simulink model "SystemPIDOpenLoopTest"  (Simulink 7.7)
settings: Solver=ode4  StartTime=0.0  StopTime=50  FixedStep=0.01  RelTol=1e-3
libraries: simulink x4
settings Model: Creator=Rakhi  LastModifiedBy=Rakhi

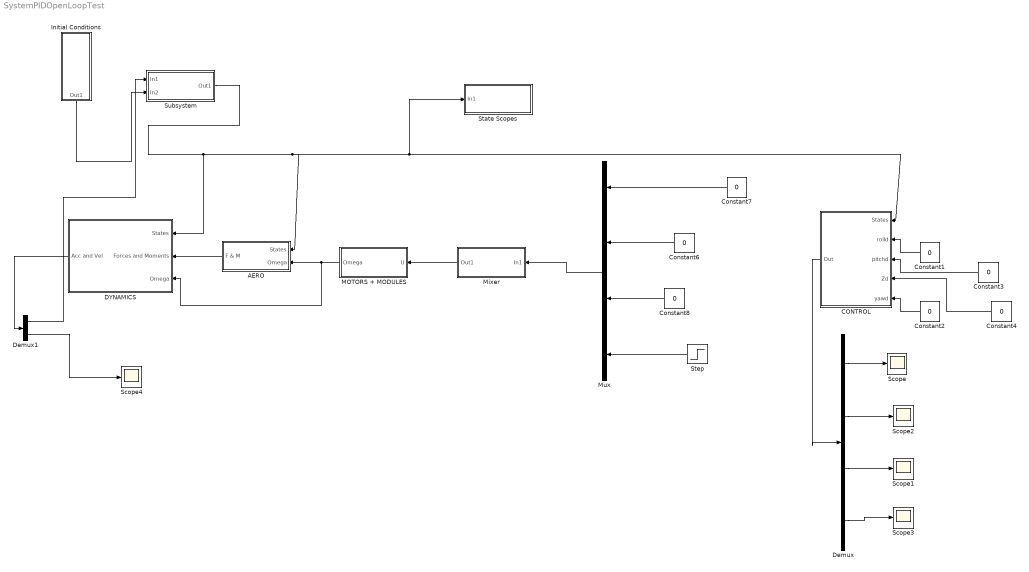
== system SystemPIDOpenLoopTest ==
  AERO : Subsystem
  CONTROL : Subsystem
  Constant{1..4,6..8} (7 alike) : Constant  Value=0
  DYNAMICS : Subsystem
  Demux : Demux
  Demux1 : Demux  Outputs=[12 1]
  Initial Conditions : Subsystem
  MOTORS + MODULES : Subsystem
  Mixer : Subsystem
  Mux : Mux
  Scope{,1..4} (5 alike) : Scope
      Scope2 settings: SaveName=ScopeData2
      Scope3 settings: SaveName=ScopeData3
      Scope4 settings: SaveName=ScopeData4
  State Scopes : Subsystem
  Step : Step  Time=10  After=-10  SampleTime=0
  Subsystem : Subsystem
  wires:
  AERO/1(F & M) -> DYNAMICS/2(Forces and Moments)
  MOTORS + MODULES/1(Omega) -> AERO/2(Omega), DYNAMICS/3(Omega)
  Constant1/1 -> CONTROL/2(rolld)
  Constant3/1 -> CONTROL/3(pitchd)
  Constant2/1 -> CONTROL/5(yawd)
  Initial Conditions/1(Out1) -> Subsystem/2(In2)
  Subsystem/1(Out1) -> DYNAMICS/1(States), AERO/1(States), CONTROL/1(States), State Scopes/1(In1)
  Mixer/1(Out1) -> MOTORS + MODULES/1(U)
  Constant4/1 -> CONTROL/4(Zd)
  Mux/1 -> Mixer/1(In1)
  Demux/1 -> Scope/1
  Demux/2 -> Scope2/1
  Demux/3 -> Scope1/1
  Demux/4 -> Scope3/1
  CONTROL/1(Out) -> Demux/1
  Demux1/1 -> Subsystem/1(In1)
  DYNAMICS/1(Acc and Vel) -> Demux1/1
  Demux1/2 -> Scope4/1
  Constant7/1 -> Mux/1
  Constant6/1 -> Mux/2
  Step/1 -> Mux/4
  Constant8/1 -> Mux/3

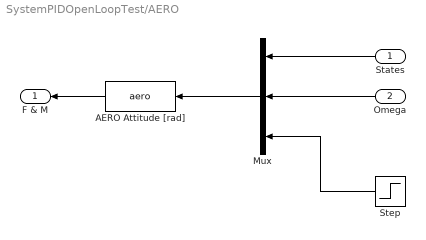
== system SystemPIDOpenLoopTest/AERO ==
  States : Inport
  Omega : Inport  Port=2
  AERO Attitude [rad] : MATLABFcn  MATLABFcn=aero  OutputDimensions=24
  Mux : Mux  Inputs=3
  Step : Step  Time=0  Before=4  After=4  SampleTime=0
  F & M : Outport
  wires:
  Step/1 -> Mux/3
  Omega/1 -> Mux/2
  States/1 -> Mux/1
  Mux/1 -> AERO Attitude [rad]/1
  AERO Attitude [rad]/1 -> F & M/1

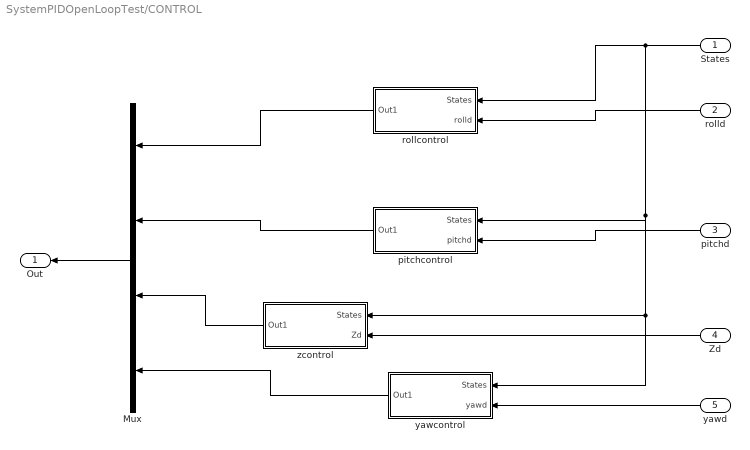
== system SystemPIDOpenLoopTest/CONTROL ==
  States : Inport
  rolld : Inport  Port=2
  pitchd : Inport  Port=3
  Zd : Inport  Port=4
  yawd : Inport  Port=5
  Mux : Mux
  pitchcontrol : Subsystem
  rollcontrol : Subsystem
  yawcontrol : Subsystem
  zcontrol : Subsystem
  Out : Outport
  wires:
  States/1 -> rollcontrol/1(States), pitchcontrol/1(States), yawcontrol/1(States), zcontrol/1(States)
  rolld/1 -> rollcontrol/2(rolld)
  pitchd/1 -> pitchcontrol/2(pitchd)
  yawd/1 -> yawcontrol/2(yawd)
  Zd/1 -> zcontrol/2(Zd)
  rollcontrol/1(Out1) -> Mux/1
  pitchcontrol/1(Out1) -> Mux/2
  zcontrol/1(Out1) -> Mux/3
  yawcontrol/1(Out1) -> Mux/4
  Mux/1 -> Out/1

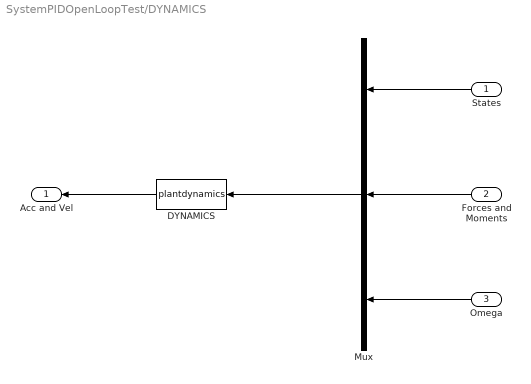
== system SystemPIDOpenLoopTest/DYNAMICS ==
  States : Inport
  Forces and Moments : Inport  Port=2
  Omega : Inport  Port=3
  DYNAMICS : MATLABFcn  MATLABFcn=plantdynamics  OutputDimensions=13
  Mux : Mux  Inputs=3
  Acc and Vel : Outport
  wires:
  States/1 -> Mux/1
  Forces and Moments/1 -> Mux/2
  Omega/1 -> Mux/3
  Mux/1 -> DYNAMICS/1
  DYNAMICS/1 -> Acc and Vel/1

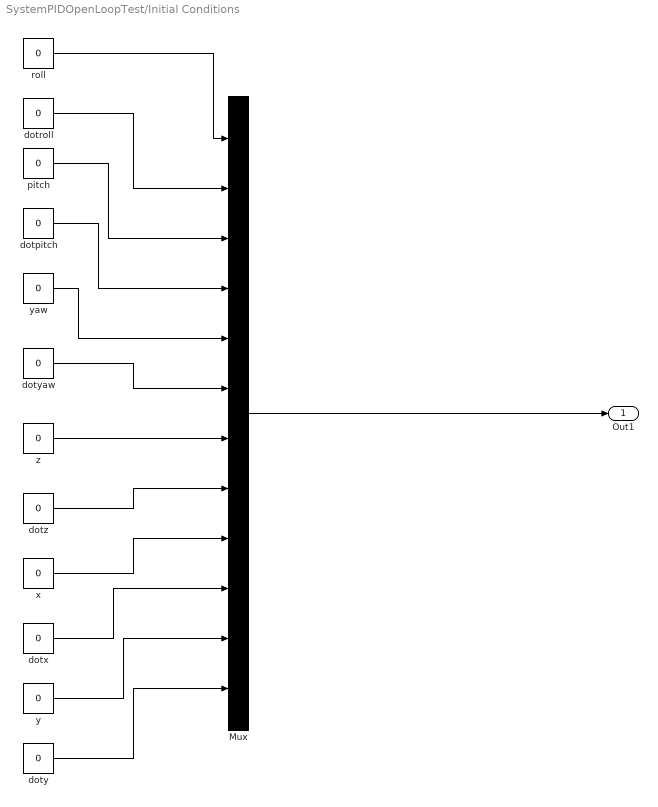
== system SystemPIDOpenLoopTest/Initial Conditions ==
  Mux : Mux  Inputs=12
  dotpitch : Constant  Value=0
  dotroll : Constant  Value=0
  dotx : Constant  Value=0
  doty : Constant  Value=0
  dotyaw : Constant  Value=0
  dotz : Constant  Value=0
  pitch : Constant  Value=0
  roll : Constant  Value=0
  x : Constant  Value=0
  y : Constant  Value=0
  yaw : Constant  Value=0
  z : Constant  Value=0
  Out1 : Outport
  wires:
  doty/1 -> Mux/12
  y/1 -> Mux/11
  dotx/1 -> Mux/10
  x/1 -> Mux/9
  dotz/1 -> Mux/8
  z/1 -> Mux/7
  dotyaw/1 -> Mux/6
  yaw/1 -> Mux/5
  dotpitch/1 -> Mux/4
  pitch/1 -> Mux/3
  dotroll/1 -> Mux/2
  roll/1 -> Mux/1
  Mux/1 -> Out1/1

== system SystemPIDOpenLoopTest/MOTORS + MODULES ==
  U : Inport
  MOTOR DYNAMICS : Subsystem
  Omega : Outport
  wires:
  U/1 -> MOTOR DYNAMICS/1(In1)
  MOTOR DYNAMICS/1(Out1) -> Omega/1

== system SystemPIDOpenLoopTest/Mixer ==
  In1 : Inport
  Interpreted MATLAB Function : MATLABFcn  MATLABFcn=mix  OutputDimensions=4
  Out1 : Outport
  wires:
  In1/1 -> Interpreted MATLAB Function/1
  Interpreted MATLAB Function/1 -> Out1/1

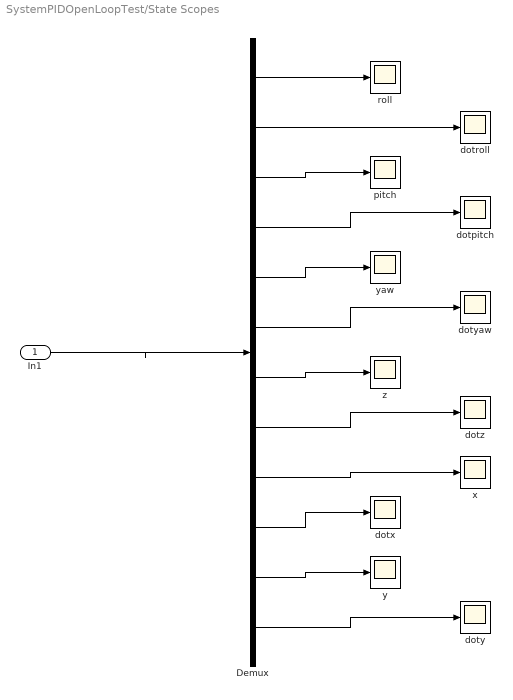
== system SystemPIDOpenLoopTest/State Scopes ==
  In1 : Inport
  Demux : Demux  Outputs=12
  dotpitch : Scope
      settings: SaveName=ScopeData8
  dotroll : Scope
      settings: SaveName=ScopeData6
  dotx : Scope
      settings: SaveName=ScopeData14
  doty : Scope
      settings: SaveName=ScopeData16
  dotyaw : Scope
      settings: SaveName=ScopeData10
  dotz : Scope
      settings: SaveName=ScopeData12
  pitch : Scope
      settings: SaveName=ScopeData7
  roll : Scope
      settings: SaveName=ScopeData5
  x : Scope
      settings: SaveName=ScopeData13
  y : Scope
      settings: SaveName=ScopeData15
  yaw : Scope
      settings: SaveName=ScopeData9
  z : Scope
      settings: SaveName=ScopeData11
  wires:
  In1/1 -> Demux/1
  Demux/1 -> roll/1
  Demux/2 -> dotroll/1
  Demux/3 -> pitch/1
  Demux/4 -> dotpitch/1
  Demux/5 -> yaw/1
  Demux/6 -> dotyaw/1
  Demux/7 -> z/1
  Demux/8 -> dotz/1
  Demux/9 -> x/1
  Demux/10 -> dotx/1
  Demux/11 -> y/1
  Demux/12 -> doty/1

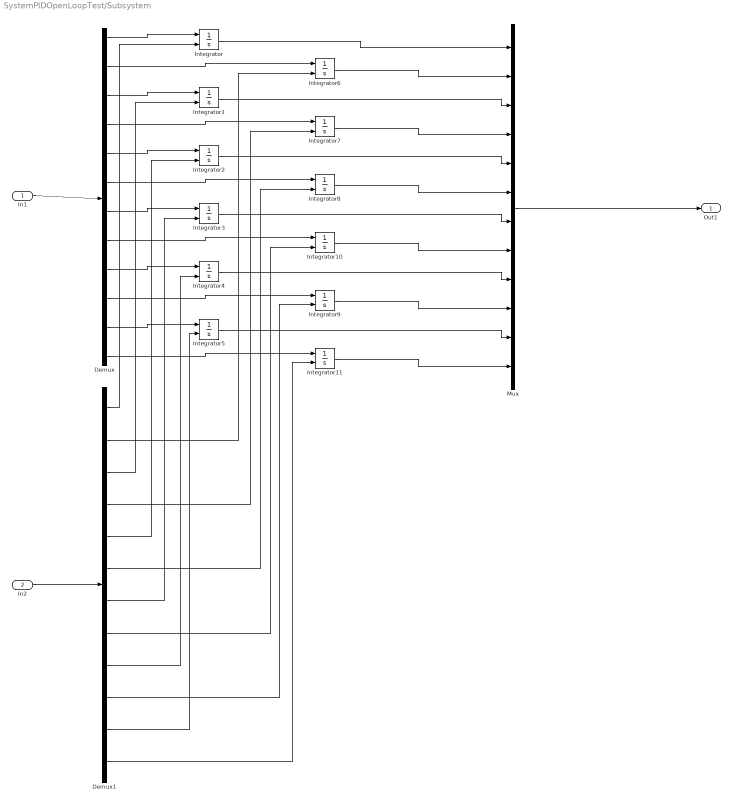
== system SystemPIDOpenLoopTest/Subsystem ==
  In1 : Inport
  In2 : Inport  Port=2
  Demux : Demux  Outputs=12
  Demux1 : Demux  Outputs=12
  Integrator{,1..11} (12 alike) : Integrator  InitialConditionSource=external
  Mux : Mux  Inputs=12
  Out1 : Outport
  wires:
  Demux/1 -> Integrator/1
  Demux/2 -> Integrator6/1
  Demux/3 -> Integrator1/1
  Demux/4 -> Integrator7/1
  Demux/5 -> Integrator2/1
  Demux/6 -> Integrator8/1
  Demux/7 -> Integrator3/1
  Demux/8 -> Integrator10/1
  Demux/9 -> Integrator4/1
  Demux/10 -> Integrator9/1
  Demux/11 -> Integrator5/1
  Demux/12 -> Integrator11/1
  In1/1 -> Demux/1
  Demux1/1 -> Integrator/2
  Demux1/2 -> Integrator6/2
  Demux1/3 -> Integrator1/2
  Demux1/4 -> Integrator7/2
  Demux1/5 -> Integrator2/2
  Demux1/6 -> Integrator8/2
  Demux1/7 -> Integrator3/2
  Demux1/8 -> Integrator10/2
  Demux1/9 -> Integrator4/2
  Demux1/10 -> Integrator9/2
  Demux1/11 -> Integrator5/2
  Demux1/12 -> Integrator11/2
  In2/1 -> Demux1/1
  Integrator/1 -> Mux/1
  Integrator6/1 -> Mux/2
  Integrator1/1 -> Mux/3
  Integrator7/1 -> Mux/4
  Integrator2/1 -> Mux/5
  Integrator8/1 -> Mux/6
  Integrator3/1 -> Mux/7
  Integrator10/1 -> Mux/8
  Integrator4/1 -> Mux/9
  Integrator9/1 -> Mux/10
  Integrator5/1 -> Mux/11
  Integrator11/1 -> Mux/12
  Mux/1 -> Out1/1

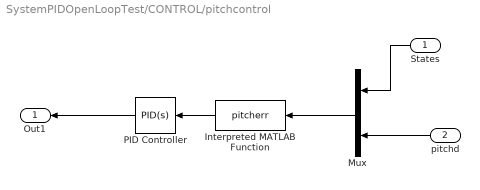
== system SystemPIDOpenLoopTest/CONTROL/pitchcontrol ==
  States : Inport
  pitchd : Inport  Port=2
  Interpreted MATLAB Function : MATLABFcn  MATLABFcn=pitcherr  OutputDimensions=1
  Mux : Mux  Inputs=2
  PID Controller : simulink/Continuous/PID Controller  SystemSampleTime=-1  Controller=PID  TimeDomain=Continuous-time  SampleTime=1  IntegratorMethod=Forward Euler  FilterMethod=Forward Euler  Form=Parallel  P=1  I=1  D=0  N=100  InitialConditionSource=internal  InitialConditionForIntegrator=0  InitialConditionForFilter=0  ExternalReset=none  LimitOutput=off  UpperSaturationLimit=inf  LowerSaturationLimit=-inf  LinearizeAsGain=off  AntiWindupMode=none  Kb=1  TrackingMode=off  Kt=1  PParamMin=[]  PParamMax=[]  IParamMin=[]  IParamMax=[]  DParamMin=[]  DParamMax=[]  NParamMin=[]  NParamMax=[]  KbParamMin=[]  KbParamMax=[]  KtParamMin=[]  KtParamMax=[]  POutMin=[]  POutMax=[]  IOutMin=[]  IOutMax=[]  DOutMin=[]  DOutMax=[]  NOutMin=[]  NOutMax=[]  KbOutMin=[]  KbOutMax=[]  KtOutMin=[]  KtOutMax=[]  IntegratorOutMin=[]  IntegratorOutMax=[]  FilterOutMin=[]  FilterOutMax=[]  SumOutMin=[]  SumOutMax=[]  SumI1OutMin=[]  SumI1OutMax=[]  SumI2OutMin=[]  SumI2OutMax=[]  SumI3OutMin=[]  SumI3OutMax=[]  SumDOutMin=[]  SumDOutMax=[]  SaturationOutMin=[]  SaturationOutMax=[]  IntegratorContinuousStateAttributes=''  IntegratorStateMustResolveToSignalObject=off  IntegratorRTWStateStorageClass=Auto  FilterContinuousStateAttributes=''  FilterStateMustResolveToSignalObject=off  FilterRTWStateStorageClass=Auto
  Out1 : Outport
  wires:
  States/1 -> Mux/1
  pitchd/1 -> Mux/2
  Mux/1 -> Interpreted MATLAB Function/1
  Interpreted MATLAB Function/1 -> PID Controller/1
  PID Controller/1 -> Out1/1

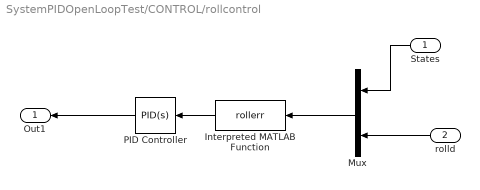
== system SystemPIDOpenLoopTest/CONTROL/rollcontrol ==
  States : Inport
  rolld : Inport  Port=2
  Interpreted MATLAB Function : MATLABFcn  MATLABFcn=rollerr  OutputDimensions=1
  Mux : Mux  Inputs=2
  PID Controller : simulink/Continuous/PID Controller  SystemSampleTime=-1  Controller=PID  TimeDomain=Continuous-time  SampleTime=1  IntegratorMethod=Forward Euler  FilterMethod=Forward Euler  Form=Parallel  P=1  I=1  D=0  N=100  InitialConditionSource=internal  InitialConditionForIntegrator=0  InitialConditionForFilter=0  ExternalReset=none  LimitOutput=off  UpperSaturationLimit=inf  LowerSaturationLimit=-inf  LinearizeAsGain=off  AntiWindupMode=none  Kb=1  TrackingMode=off  Kt=1  PParamMin=[]  PParamMax=[]  IParamMin=[]  IParamMax=[]  DParamMin=[]  DParamMax=[]  NParamMin=[]  NParamMax=[]  KbParamMin=[]  KbParamMax=[]  KtParamMin=[]  KtParamMax=[]  POutMin=[]  POutMax=[]  IOutMin=[]  IOutMax=[]  DOutMin=[]  DOutMax=[]  NOutMin=[]  NOutMax=[]  KbOutMin=[]  KbOutMax=[]  KtOutMin=[]  KtOutMax=[]  IntegratorOutMin=[]  IntegratorOutMax=[]  FilterOutMin=[]  FilterOutMax=[]  SumOutMin=[]  SumOutMax=[]  SumI1OutMin=[]  SumI1OutMax=[]  SumI2OutMin=[]  SumI2OutMax=[]  SumI3OutMin=[]  SumI3OutMax=[]  SumDOutMin=[]  SumDOutMax=[]  SaturationOutMin=[]  SaturationOutMax=[]  IntegratorContinuousStateAttributes=''  IntegratorStateMustResolveToSignalObject=off  IntegratorRTWStateStorageClass=Auto  FilterContinuousStateAttributes=''  FilterStateMustResolveToSignalObject=off  FilterRTWStateStorageClass=Auto
  Out1 : Outport
  wires:
  States/1 -> Mux/1
  rolld/1 -> Mux/2
  Mux/1 -> Interpreted MATLAB Function/1
  Interpreted MATLAB Function/1 -> PID Controller/1
  PID Controller/1 -> Out1/1

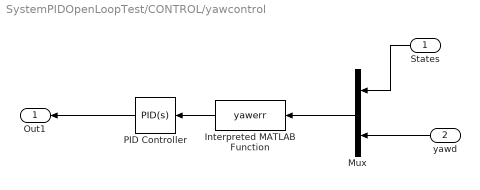
== system SystemPIDOpenLoopTest/CONTROL/yawcontrol ==
  States : Inport
  yawd : Inport  Port=2
  Interpreted MATLAB Function : MATLABFcn  MATLABFcn=yawerr  OutputDimensions=1
  Mux : Mux  Inputs=2
  PID Controller : simulink/Continuous/PID Controller  SystemSampleTime=-1  Controller=PID  TimeDomain=Continuous-time  SampleTime=1  IntegratorMethod=Forward Euler  FilterMethod=Forward Euler  Form=Parallel  P=1  I=1  D=0  N=100  InitialConditionSource=internal  InitialConditionForIntegrator=0  InitialConditionForFilter=0  ExternalReset=none  LimitOutput=off  UpperSaturationLimit=inf  LowerSaturationLimit=-inf  LinearizeAsGain=off  AntiWindupMode=none  Kb=1  TrackingMode=off  Kt=1  PParamMin=[]  PParamMax=[]  IParamMin=[]  IParamMax=[]  DParamMin=[]  DParamMax=[]  NParamMin=[]  NParamMax=[]  KbParamMin=[]  KbParamMax=[]  KtParamMin=[]  KtParamMax=[]  POutMin=[]  POutMax=[]  IOutMin=[]  IOutMax=[]  DOutMin=[]  DOutMax=[]  NOutMin=[]  NOutMax=[]  KbOutMin=[]  KbOutMax=[]  KtOutMin=[]  KtOutMax=[]  IntegratorOutMin=[]  IntegratorOutMax=[]  FilterOutMin=[]  FilterOutMax=[]  SumOutMin=[]  SumOutMax=[]  SumI1OutMin=[]  SumI1OutMax=[]  SumI2OutMin=[]  SumI2OutMax=[]  SumI3OutMin=[]  SumI3OutMax=[]  SumDOutMin=[]  SumDOutMax=[]  SaturationOutMin=[]  SaturationOutMax=[]  IntegratorContinuousStateAttributes=''  IntegratorStateMustResolveToSignalObject=off  IntegratorRTWStateStorageClass=Auto  FilterContinuousStateAttributes=''  FilterStateMustResolveToSignalObject=off  FilterRTWStateStorageClass=Auto
  Out1 : Outport
  wires:
  States/1 -> Mux/1
  yawd/1 -> Mux/2
  Mux/1 -> Interpreted MATLAB Function/1
  Interpreted MATLAB Function/1 -> PID Controller/1
  PID Controller/1 -> Out1/1

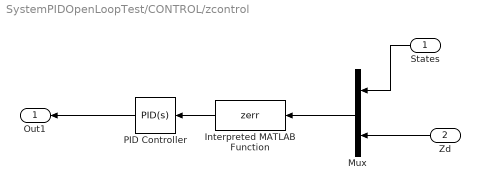
== system SystemPIDOpenLoopTest/CONTROL/zcontrol ==
  States : Inport
  Zd : Inport  Port=2
  Interpreted MATLAB Function : MATLABFcn  MATLABFcn=zerr  OutputDimensions=1
  Mux : Mux  Inputs=2
  PID Controller : simulink/Continuous/PID Controller  SystemSampleTime=-1  Controller=PID  TimeDomain=Continuous-time  SampleTime=1  IntegratorMethod=Forward Euler  FilterMethod=Forward Euler  Form=Parallel  P=1  I=1  D=0  N=100  InitialConditionSource=internal  InitialConditionForIntegrator=0  InitialConditionForFilter=0  ExternalReset=none  LimitOutput=off  UpperSaturationLimit=inf  LowerSaturationLimit=-inf  LinearizeAsGain=off  AntiWindupMode=none  Kb=1  TrackingMode=off  Kt=1  PParamMin=[]  PParamMax=[]  IParamMin=[]  IParamMax=[]  DParamMin=[]  DParamMax=[]  NParamMin=[]  NParamMax=[]  KbParamMin=[]  KbParamMax=[]  KtParamMin=[]  KtParamMax=[]  POutMin=[]  POutMax=[]  IOutMin=[]  IOutMax=[]  DOutMin=[]  DOutMax=[]  NOutMin=[]  NOutMax=[]  KbOutMin=[]  KbOutMax=[]  KtOutMin=[]  KtOutMax=[]  IntegratorOutMin=[]  IntegratorOutMax=[]  FilterOutMin=[]  FilterOutMax=[]  SumOutMin=[]  SumOutMax=[]  SumI1OutMin=[]  SumI1OutMax=[]  SumI2OutMin=[]  SumI2OutMax=[]  SumI3OutMin=[]  SumI3OutMax=[]  SumDOutMin=[]  SumDOutMax=[]  SaturationOutMin=[]  SaturationOutMax=[]  IntegratorContinuousStateAttributes=''  IntegratorStateMustResolveToSignalObject=off  IntegratorRTWStateStorageClass=Auto  FilterContinuousStateAttributes=''  FilterStateMustResolveToSignalObject=off  FilterRTWStateStorageClass=Auto
  Out1 : Outport
  wires:
  States/1 -> Mux/1
  Zd/1 -> Mux/2
  Mux/1 -> Interpreted MATLAB Function/1
  Interpreted MATLAB Function/1 -> PID Controller/1
  PID Controller/1 -> Out1/1

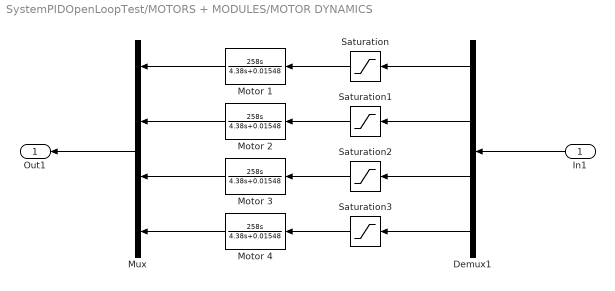
== system SystemPIDOpenLoopTest/MOTORS + MODULES/MOTOR DYNAMICS ==
  In1 : Inport
  Demux1 : Demux
  Motor {1..4} (4 alike) : TransferFcn  Numerator=[258 0]  Denominator=[4.38 0.01548]
  Mux : Mux
  Saturation{,1..3} (4 alike) : Saturate  UpperLimit=250  LowerLimit=-250
  Out1 : Outport
  wires:
  In1/1 -> Demux1/1
  Demux1/1 -> Saturation/1
  Demux1/2 -> Saturation1/1
  Demux1/3 -> Saturation2/1
  Demux1/4 -> Saturation3/1
  Mux/1 -> Out1/1
  Motor 2/1 -> Mux/2
  Motor 3/1 -> Mux/3
  Motor 4/1 -> Mux/4
  Motor 1/1 -> Mux/1
  Saturation/1 -> Motor 1/1
  Saturation1/1 -> Motor 2/1
  Saturation2/1 -> Motor 3/1
  Saturation3/1 -> Motor 4/1
